simulink model "geo_affine"  (Simulink 8.3)
settings: Solver=FixedStepDiscrete  StartTime=0.0  StopTime=5  RelTol=1e-3
undefined symbols (not defined in the file or in its folder): gray
libraries: visionsinks x2, visiongeotforms x1, visionsources x1
settings Model: Creator=FxMain  LastModifiedBy=Vasilis
settings DataIOCC: InspectSignalLogs=on
settings OptimizationCC: ExpressionDepthLimit=2147483647
settings DebuggingCC: FcnCallInpInsideContextMsg=UseLocalSettings

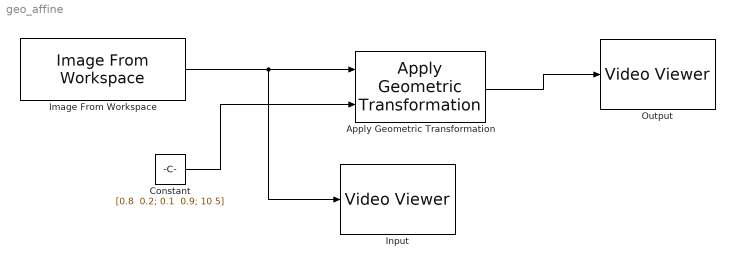
== system geo_affine ==
  Apply Geometric Transformation : visiongeotforms/Apply Geometric Transformation  tformSource=Input port  tformValue=[1 0 0; 0 1 0; 0 0 1]  approxProjectiveFlag=off  errorTolerance=1.0  roiMethod=Whole input image  roiSource=Specify via dialog  roiBBox=[1 1 256 128]  roiVertice=[1 1 12 10 22 20]  inputClipFlag=off  interpolationMethod=Bilinear  fillValue=0  viewPortMethod=Same as input image  outputSize=[512 512]  outputLoc=[1 1]  outputClipFlag=off
  Constant : Constant  Value="[0.8  0.2; 0.1  0.9; 10 5]"  VectorParams1D=off
      settings: SamplingMode=Frame based
  Image From Workspace : visionsources/Image From Workspace  Tag=vipblks_nd  ImageValue=img  Ts=inf  imagePorts=One multidimensional signal  ImageDataType=Inherit from 'Value'  Signed=on  WordLength=16  sdImageDataType=sfix(16)  FractionLengthMode=User-defined  FractionLength=15  OutPortLabels=R|G|B
  Input : visionsinks/Video Viewer  inputType=Obsolete7b  imagePorts=One multidimensional signal  useColorMap=off  colormapValue=gray(256)  specRange=on  minInputVal=0  maxInputVal=255  FigPos=[78 797 838 674]  AxisZoom=on  trueSizedOnce=off  OpenAtMdlStart=on  DefaultConfigurationName=vipscopes.VideoViewerScopeCfg
  Output : visionsinks/Video Viewer  inputType=Obsolete7b  imagePorts=One multidimensional signal  useColorMap=off  colormapValue=gray(256)  specRange=on  minInputVal=0  maxInputVal=255  FigPos=[1640 807 628 558]  AxisZoom=on  trueSizedOnce=off  OpenAtMdlStart=on  DefaultConfigurationName=vipscopes.VideoViewerScopeCfg
  wires:
  Apply Geometric Transformation/1 -> Output/1
  Constant/1 -> Apply Geometric Transformation/2
  Image From Workspace/1 -> Input/1, Apply Geometric Transformation/1
